simulink model "AMsimulation"  (R2016a)
settings: Solver=ode3  SolverMode=SingleTasking  StartTime=0.0  StopTime=inf  RelTol=1e-3
libraries: dsparch4 x2
settings Model: Creator=THINKPAD  LastModifiedBy=THINKPAD
settings SolverCC: AutoInsertRateTranBlk=on
settings DataIOCC: LimitDataPoints=on  SaveOutput=off  SignalLogging=off  SaveTime=off
settings DebuggingCC: AlgebraicLoopMsg=error  SingleTaskRateTransMsg=error  AllowSymbolicDim=off

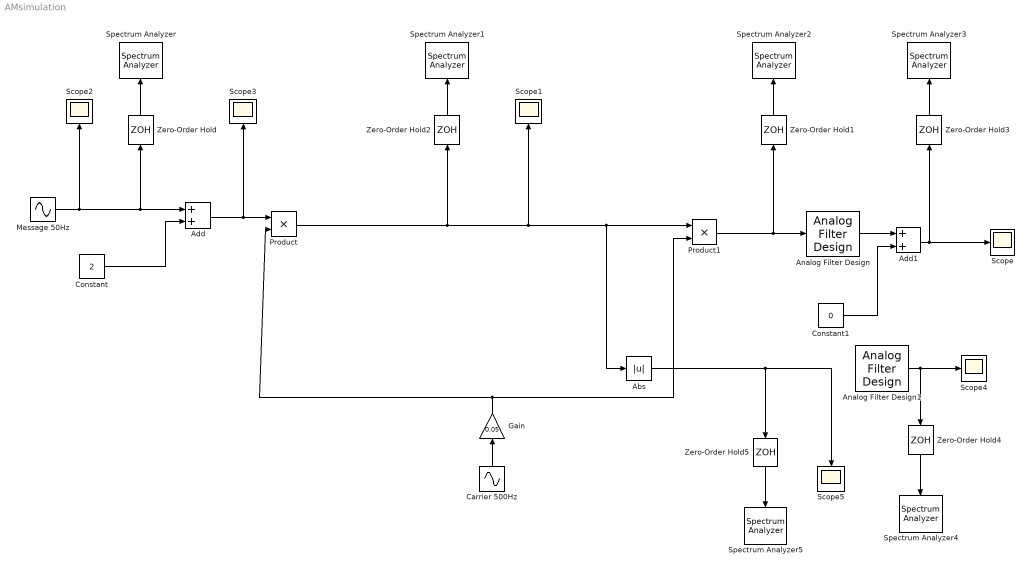
== system AMsimulation ==
  Abs : Abs
  Add : Sum
  Add1 : Sum
  Analog Filter Design : dsparch4/Analog Filter Design  method=Butterworth  filttype=Lowpass  N=8  Wlo=15*pi  Whi=80  Rp=2  Rs=40
  Analog Filter Design1 : dsparch4/Analog Filter Design  method=Butterworth  filttype=Lowpass  N=8  Wlo=15*pi  Whi=80  Rp=2  Rs=40
  Carrier 500Hz : Sin  Frequency=100*pi  SampleTime=0
  Constant : Constant  Value=2
  Constant1 : Constant  Value=0
  Gain : Gain  Gain=0.05
  Message 50Hz : Sin  Frequency=10*pi  Samples=5  SampleTime=0
  Product : Product
  Product1 : Product
  Scope{,1..5} (6 alike) : Scope
  Spectrum Analyzer{,1..5} (6 alike) : SpectrumAnalyzer
  Zero-Order Hold : ZeroOrderHold  SampleTime=1/150
  Zero-Order Hold{1..5} (5 alike) : ZeroOrderHold  SampleTime=1/1500
  wires:
  Constant/1 -> Add/2
  Add/1 -> Scope3/1, Product/1
  Carrier 500Hz/1 -> Gain/1
  Product/1 -> Scope1/1, Abs/1, Product1/1, Zero-Order Hold2/1
  Zero-Order Hold/1 -> Spectrum Analyzer/1
  Zero-Order Hold2/1 -> Spectrum Analyzer1/1
  Product1/1 -> Analog Filter Design/1, Zero-Order Hold1/1
  Zero-Order Hold1/1 -> Spectrum Analyzer2/1
  Zero-Order Hold3/1 -> Spectrum Analyzer3/1
  Analog Filter Design/1 -> Add1/1
  Constant1/1 -> Add1/2
  Add1/1 -> Scope/1, Zero-Order Hold3/1
  Message 50Hz/1 -> Scope2/1, Add/1, Zero-Order Hold/1
  Gain/1 -> Product/2, Product1/2
  Zero-Order Hold4/1 -> Spectrum Analyzer4/1
  Analog Filter Design1/1 -> Scope4/1, Zero-Order Hold4/1
  Zero-Order Hold5/1 -> Spectrum Analyzer5/1
  Abs/1 -> Scope5/1, Zero-Order Hold5/1
